simulink model "untitled1"  (R2013a)
settings: Solver=ode45  StartTime=0.0  StopTime=100.0  RelTol=1e-6
settings Model: Creator=David  LastModifiedBy=David

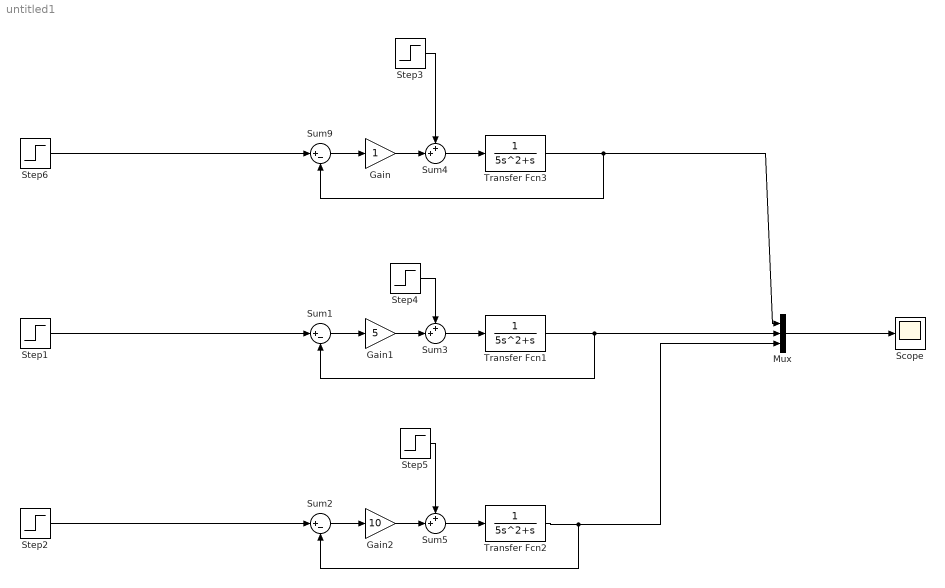
== system untitled1 ==
  Gain : Gain
  Gain1 : Gain  Gain=5
  Gain2 : Gain  Gain=10
  Mux : Mux  Inputs=3
  Scope : Scope
  Step1 : Step  SampleTime=0
  Step2 : Step  SampleTime=0
  Step3 : Step  Before=-0.3  SampleTime=0
  Step4 : Step  Before=-0.3  SampleTime=0
  Step5 : Step  Before=-0.3  SampleTime=0
  Step6 : Step  SampleTime=0
  Sum1 : Sum  Inputs=|+-
  Sum2 : Sum  Inputs=|+-
  Sum3 : Sum  Inputs=++|
  Sum4 : Sum  Inputs=++|
  Sum5 : Sum  Inputs=++|
  Sum9 : Sum  Inputs=|+-
  Transfer Fcn1 : TransferFcn  Denominator=[5 1 0]
  Transfer Fcn2 : TransferFcn  Denominator=[5 1 0]
  Transfer Fcn3 : TransferFcn  Denominator=[5 1 0]
  wires:
  Transfer Fcn3/1 -> Sum9/2, Mux/1
  Sum9/1 -> Gain/1
  Step6/1 -> Sum9/1
  Transfer Fcn1/1 -> Mux/2, Sum1/2
  Sum1/1 -> Gain1/1
  Step1/1 -> Sum1/1
  Transfer Fcn2/1 -> Mux/3, Sum2/2
  Sum2/1 -> Gain2/1
  Step2/1 -> Sum2/1
  Mux/1 -> Scope/1
  Sum5/1 -> Transfer Fcn2/1
  Gain2/1 -> Sum5/2
  Sum4/1 -> Transfer Fcn3/1
  Gain/1 -> Sum4/2
  Sum3/1 -> Transfer Fcn1/1
  Gain1/1 -> Sum3/2
  Step5/1 -> Sum5/1
  Step4/1 -> Sum3/1
  Step3/1 -> Sum4/1
